simulink model "SimulinkRobot_Test2_PDandGravityComp"  (R2023b)
settings: Solver=VariableStepAuto  StartTime=0.0  StopTime=10  RelTol=1e-3
values from neighbouring files (symbols this model uses):
  grav = [0;0;0;0;0;-9.8]    [regressorTest.m]
undefined symbols (not defined in the file or in its folder): Mlist, TfLists, Twists
libraries: slpidlib x1
settings Model: Creator=mechmedic  LastModifiedBy=mechmedic

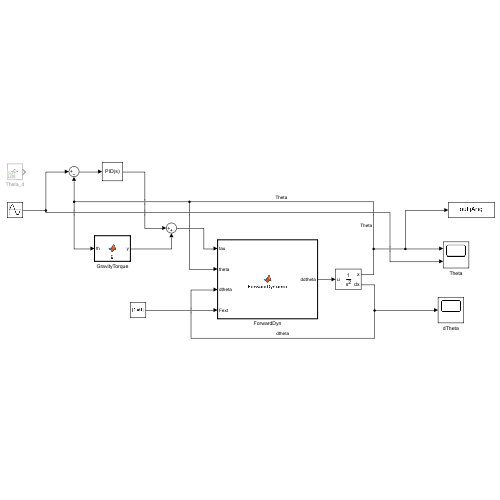
[thumbnail: Simulink's stored preview of the top-level diagram]
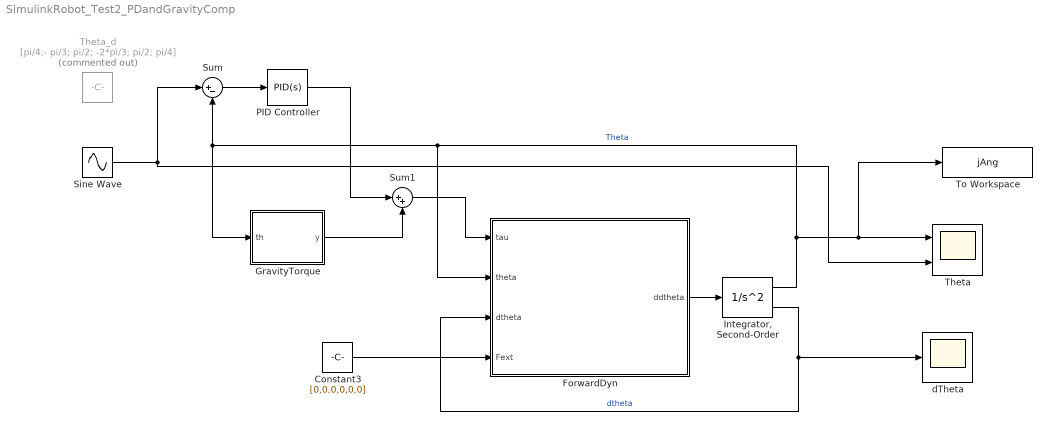
== system SimulinkRobot_Test2_PDandGravityComp ==
  Constant3 : Constant  Value=[0,0,0,0,0,0]
  ForwardDyn : MATLAB Function  TreatAsAtomicUnit=on
  GravityTorque : MATLAB Function  TreatAsAtomicUnit=on
  "Integrator, Second-Order" : SecondOrderIntegrator
  PID Controller : slpidlib/PID Controller  Controller=PID  Form=Parallel  TimeDomain=Continuous-time  UseExternalTs=off  SampleTime=-1  IntegratorMethod=Forward Euler  FilterMethod=Forward Euler  ControllerParametersSource=internal  P=30  I=0  UseKiTs=off  D=10  N=100  UseFilter=on  TunerSelectOption=Transfer Function Based (PID Tuner App)  InitialConditionSource=internal  InitialConditionForIntegrator=0  InitialConditionForFilter=0  DifferentiatorICPrevScaledInput=0  ExternalReset=none  TrackingMode=off  Kt=1  LimitOutput=off  SatLimitsSource=internal  UpperSaturationLimit=inf  LowerSaturationLimit=-inf  LinearizeAsGain=on  AntiWindupMode=none  Kb=1  LimitIntegrator=off  UpperIntegratorSaturationLimit=inf  LowerIntegratorSaturationLimit=-inf  POutMin=[]  POutMax=[]  IOutMin=[]  IOutMax=[]  DOutMin=[]  DOutMax=[]  NOutMin=[]  NOutMax=[]  SumOutMin=[]  SumOutMax=[]  SaturationOutMin=[]  SaturationOutMax=[]  PParamMin=[]  PParamMax=[]  IParamMin=[]  IParamMax=[]  DParamMin=[]  DParamMax=[]  NParamMin=[]  NParamMax=[]  KbParamMin=[]  KbParamMax=[]  KtParamMin=[]  KtParamMax=[]  KbOutMin=[]  KbOutMax=[]  KtOutMin=[]  KtOutMax=[]  IntegratorOutMin=[]  IntegratorOutMax=[]  FilterOutMin=[]  FilterOutMax=[]  SumI1OutMin=[]  SumI1OutMax=[]  SumI2OutMin=[]  SumI2OutMax=[]  SumI3OutMin=[]  SumI3OutMax=[]  SumI4OutMin=[]  SumI4OutMax=[]  SumDOutMin=[]  SumDOutMax=[]  DifferentiatorOutMin=[]  DifferentiatorOutMax=[]  FilterDiffOutCoefMin=[]  FilterDiffOutCoefMax=[]  ReciprocalOutMin=[]  ReciprocalOutMax=[]  SumDenOutMin=[]  SumDenOutMax=[]  SumNumOutMin=[]  SumNumOutMax=[]  DivideOutMin=[]  DivideOutMax=[]  UdiffTsProdOutMin=[]  UdiffTsProdOutMax=[]  NTsProdOutMin=[]  NTsProdOutMax=[]  UintegralTsProdOutMin=[]  UintegralTsProdOutMax=[]  UngainTsProdOutMin=[]  UngainTsProdOutMax=[]  ClampingZeroOutDataTypeStr=Inherit: Inherit via back propagation  ClampingZeroOutMin=[]  ClampingZeroOutMax=[]  FilterDenConstantOutDataTypeStr=Inherit: Inherit via back propagation  FilterDenConstantOutMin=[]  FilterDenConstantOutMax=[]  PCopyOutDataTypeStr=Inherit: Inherit via back propagation  PCopyOutMin=[]  PCopyOutMax=[]  NCopyOutDataTypeStr=Inherit: Inherit via back propagation  NCopyOutMin=[]  NCopyOutMax=[]  IntegratorContinuousStateAttributes=''  IntegratorStateMustResolveToSignalObject=off  IntegratorRTWStateStorageClass=Auto  FilterContinuousStateAttributes=''  FilterStateMustResolveToSignalObject=off  FilterRTWStateStorageClass=Auto  ParallelPVariant=InternalParameters  IdealPVariant=Disabled  IVariant=InternalParameters  DVariant=InternalParameters  IntegratorVariant=Continuous  SatVariant=Disabled  AWVariant=Passthrough  PCopyVariant=Disabled  TRVariant=Disabled  FdbkBlocksVariant=Forward  IdealPFdbkVariant=Disabled  SatFdbkVariant=Disabled  DerivativeFilterVariant=ContFilter  NVariant=InternalParameters  NCopyVariant=Disabled  FilterICVariant=InternalICsFilter  IntegratorICVariant=InternalICs  ExternalResetVariant=Disabled  TRSumVariant=Passthrough  SumFdbkVariant=Disabled  SumVariant=Sum_PID  TsampFilterVariant=InternalTs  TsampNgainVariant=Passthrough  TsampIntegralVariant=Disabled_SignalSpec  ExternalSaturationOutDataTypeStr=Inherit: Same as second input
  Sine Wave : Sin  Amplitude=[pi/3, -pi/2, pi/3, pi/2, pi/4, pi/2]  Frequency=[1, 1, 1, 1, 1, 1]  SampleTime=0
  Sum : Sum  Inputs=|+-
  Sum1 : Sum  Inputs=|++
  Theta : Scope  NumInputPorts=2
  Theta_d : Constant  Commented=on  Value=[pi/4;- pi/3; pi/2; -2*pi/3; pi/2; pi/4]
  To Workspace : ToWorkspace  VariableName=jAng  SaveFormat=Timeseries  SampleTime=-1
  dTheta : Scope
  wires:
  Constant3/1 -> ForwardDyn/4(Fext)
  ForwardDyn/1(ddtheta) -> "Integrator, Second-Order"/1
  "Integrator, Second-Order"/1 -> ForwardDyn/2(theta), GravityTorque/1(th), Sum/2, To Workspace/1, Theta/1  "Theta"
  "Integrator, Second-Order"/2 -> dTheta/1, ForwardDyn/3(dtheta)  "dtheta"
  GravityTorque/1(y) -> Sum1/2
  Sum/1 -> PID Controller/1
  PID Controller/1 -> Sum1/1
  Sum1/1 -> ForwardDyn/1(tau)
  Sine Wave/1 -> Sum/1, Theta/2

== matlab function SimulinkRobot_Test2_PDandGravityComp/GravityTorque ==
  data: th input; y output; Twists parameter; TfLists parameter; Mlist parameter; grav parameter
function y = g(th,Twists, TfLists, Mlist, grav)
    y = GravityTorque(th, Twists, TfLists, Mlist, grav);

== matlab function SimulinkRobot_Test2_PDandGravityComp/ForwardDyn ==
  settings: sampleTime=0.01
  data: tau input size=[6 1]; theta input double size=[6 1]; dtheta input double size=[6 1]; Fext input; Twists parameter size=size(Twists); TfLists parameter size=size(TfLists); ddtheta output double size=[6 1]; Mlist parameter size=size(Mlist); grav parameter size=size(grav)
function ddtheta =  ForwardDynamic (tau, theta, dtheta, Fext, Twists, TfLists, Mlist, grav)
    ddtheta =  FwdDyn(tau, theta, dtheta, Fext, Twists, TfLists, Mlist, grav);
